simulink model "combfilter_org"  (Simulink 10.0)
settings: Solver=FixedStepDiscrete  StartTime=0.0  StopTime=4  RelTol=1e-3
Description:
  | Data Typing Filter
  | 
  | This example shows how a filter can be applied to signals of different
  | data types using standard Simulink(R) blocks.  In this example, a signal with
  | some noise on it is produced.  This signal is then fed into a filter as a single
  | precision data type and a standard double data type. The output from the
  | filter for each signal is then compared and the error is displayed on the
  | scope.
settings Model: Creator=The MathWorks, Inc.  LastModifiedBy=bhisma  ExtModeTrigMode=oneshot  ExtModeArmWhenConnect=off  ExtModeAutoUpdateStatusClock=off
settings DataIOCC: SaveFormat=Structure  ReturnWorkspaceOutputs=on
settings OptimizationCC: BlockReduction=off  BooleanDataType=off  InitFltsAndDblsToZero=on  BufferReusableBoundary=off
settings DebuggingCC: SaveWithParameterizedLinksMsg=none  UnderspecifiedInitializationDetection=Simplified  MergeDetectMultiDrivingBlocksExec=error  SignalResolutionControl=TryResolveAllWithWarning  MultiTaskDSMMsg=warning  MultiTaskCondExecSysMsg=none  FcnCallInpInsideContextMsg=warning  BusObjectLabelMismatch=none  AllowSymbolicDim=off  StateNameClashWarn=warning
settings HardwareCC: TargetUnknown=on
settings GRTTargetCC: TargetFcnLib=ansi_tfl_tmw.mat  GeneratePreprocessorConditionals=Disable all
settings ConfigComp: CovExternalEMLEnable=off

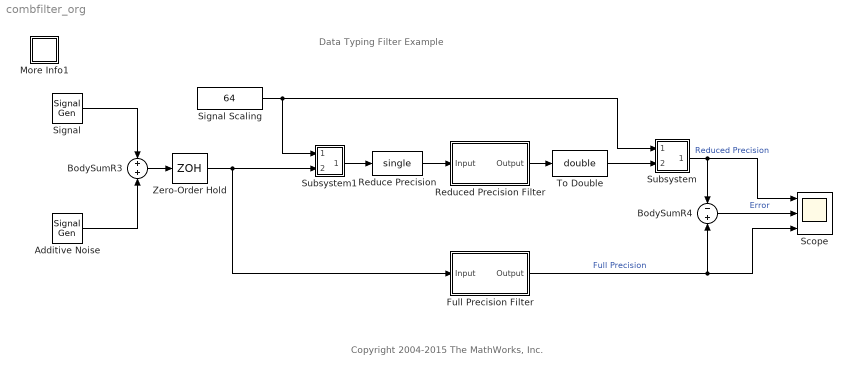
== system combfilter_org ==
  note: Data Typing Filter Example
  note: Copyright 2004-2015 The MathWorks, Inc.
  Additive Noise : SignalGenerator  Amplitude=3  Frequency=25
      settings: AttributesFormatString=Waveform: %<Waveform>\nAmplitude: %<Amplitude>\nFreq: %<Frequency> %<Units>
  BodySumR3 : Sum  SaturateOnIntegerOverflow=on  InputSameDT=on  OutDataTypeStr=Inherit: Same as first input
  BodySumR4 : Sum  Inputs=-+  SaturateOnIntegerOverflow=on  InputSameDT=on  OutDataTypeStr=Inherit: Same as first input
  Full Precision Filter : Subsystem
  More Info1 : Subsystem
      settings: OpenFcn=showdemo(bdroot(gcs))
      mask Display: disp('?')
  Reduce Precision : DataTypeConversion  OutDataTypeStr=single  SaturateOnIntegerOverflow=on  RndMeth=Zero
  Reduced Precision Filter : Subsystem
  Scope : Scope  NumInputPorts=3
  Signal : SignalGenerator  Amplitude=100
      settings: AttributesFormatString=Waveform: %<Waveform>\nAmplitude: %<Amplitude>\nFreq: %<Frequency> %<Units>
  Signal Scaling : Constant  Value=64
  Subsystem : Subsystem
      mask Display:
      | port_label('input',1,'/')
      | port_label('input',2,'x')
  Subsystem1 : Subsystem
      mask Display: disp('X')
  To Double : DataTypeConversion  OutDataTypeStr=double  SaturateOnIntegerOverflow=on  RndMeth=Zero
  Zero-Order Hold : ZeroOrderHold  SampleTime=0.01
  wires:
  Reduced Precision Filter/1(Output) -> To Double/1
  Subsystem1/1(Out1) -> Reduce Precision/1
  To Double/1 -> Subsystem/2(In2)
  Zero-Order Hold/1 -> Subsystem1/2(In2), Full Precision Filter/1(Input)
  Subsystem/1(Out1) -> Scope/1, BodySumR4/1  "Reduced Precision"
  Reduce Precision/1 -> Reduced Precision Filter/1(Input)
  Signal Scaling/1 -> Subsystem/1(In1), Subsystem1/1(In1)
  Signal/1 -> BodySumR3/1
  Additive Noise/1 -> BodySumR3/2
  BodySumR3/1 -> Zero-Order Hold/1
  BodySumR4/1 -> Scope/2  "Error"
  Full Precision Filter/1(Output) -> Scope/3, BodySumR4/2  "Full Precision"

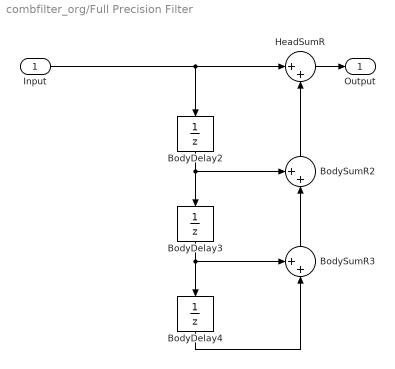
== system combfilter_org/Full Precision Filter ==
  Input : Inport
  BodyDelay2 : UnitDelay  SampleTime=-1  HasFrameUpgradeWarning=on
  BodyDelay3 : UnitDelay  SampleTime=-1  HasFrameUpgradeWarning=on
  BodyDelay4 : UnitDelay  SampleTime=-1  HasFrameUpgradeWarning=on
  BodySumR2 : Sum  Inputs=++|  SaturateOnIntegerOverflow=on  InputSameDT=on  OutDataTypeStr=Inherit: Same as first input
  BodySumR3 : Sum  Inputs=++|  SaturateOnIntegerOverflow=on  InputSameDT=on  OutDataTypeStr=Inherit: Same as first input
  HeadSumR : Sum  Inputs=|++  SaturateOnIntegerOverflow=on  InputSameDT=on  OutDataTypeStr=Inherit: Same as first input
  Output : Outport  VectorParamsAs1DForOutWhenUnconnected=off
  wires:
  Input/1 -> BodyDelay2/1, HeadSumR/1
  BodyDelay2/1 -> BodyDelay3/1, BodySumR2/1
  BodyDelay3/1 -> BodyDelay4/1, BodySumR3/1
  BodyDelay4/1 -> BodySumR3/2
  BodySumR2/1 -> HeadSumR/2
  BodySumR3/1 -> BodySumR2/2
  HeadSumR/1 -> Output/1

== system combfilter_org/More Info1 ==

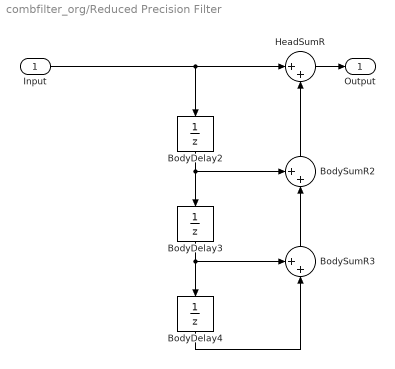
== system combfilter_org/Reduced Precision Filter ==
  Input : Inport
  BodyDelay2 : UnitDelay  SampleTime=-1  HasFrameUpgradeWarning=on
  BodyDelay3 : UnitDelay  SampleTime=-1  HasFrameUpgradeWarning=on
  BodyDelay4 : UnitDelay  SampleTime=-1  HasFrameUpgradeWarning=on
  BodySumR2 : Sum  Inputs=++|  SaturateOnIntegerOverflow=on  InputSameDT=on  OutDataTypeStr=Inherit: Same as first input
  BodySumR3 : Sum  Inputs=++|  SaturateOnIntegerOverflow=on  InputSameDT=on  OutDataTypeStr=Inherit: Same as first input
  HeadSumR : Sum  Inputs=|++  SaturateOnIntegerOverflow=on  InputSameDT=on  OutDataTypeStr=Inherit: Same as first input
  Output : Outport  VectorParamsAs1DForOutWhenUnconnected=off
  wires:
  HeadSumR/1 -> Output/1
  BodySumR3/1 -> BodySumR2/2
  BodySumR2/1 -> HeadSumR/2
  BodyDelay4/1 -> BodySumR3/2
  BodyDelay3/1 -> BodySumR3/1, BodyDelay4/1
  BodyDelay2/1 -> BodySumR2/1, BodyDelay3/1
  Input/1 -> HeadSumR/1, BodyDelay2/1

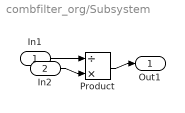
== system combfilter_org/Subsystem ==
  In1 : Inport
  In2 : Inport  Port=2
  Product : Product  Inputs=/*  SaturateOnIntegerOverflow=on  RndMeth=Zero  InputSameDT=on  OutDataTypeStr=Inherit: Same as first input
  Out1 : Outport  VectorParamsAs1DForOutWhenUnconnected=off
  wires:
  In1/1 -> Product/1
  Product/1 -> Out1/1
  In2/1 -> Product/2

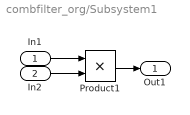
== system combfilter_org/Subsystem1 ==
  In1 : Inport
  In2 : Inport  Port=2
  Product1 : Product  SaturateOnIntegerOverflow=on  RndMeth=Zero  InputSameDT=on  OutDataTypeStr=Inherit: Same as first input
  Out1 : Outport  VectorParamsAs1DForOutWhenUnconnected=off
  wires:
  In2/1 -> Product1/2
  In1/1 -> Product1/1
  Product1/1 -> Out1/1
